simulink model "VCMGCM1962020b_v2"  (R2020b)
settings: Solver=FixedStepDiscrete  StartTime=0.0  StopTime=10.0  FixedStep=0.005  RelTol=1e-3  EnableMultiTasking=on
PreLoadFcn:
  | try, model_open; catch, disp('Error occurred while executing model pre-load callback: model_open.m'); disp('Please assure that the MATLAB working directory is set to the model directory before opening.'); end
InitFcn:
  | try, model_open; catch, end
undefined symbols (not defined in the file): Bridge, GCM, H, raptor_get_param_eval, raptor_get_safe_string, raptor_xcp_function
libraries: Blocks_lib x1165, Raptor_lib x665, simulink x62, VCM_lib x5
(part 10 of 23)

== system VCMGCM1962020b_v2/Fgnd/Diagnostics/Fault Statuses/Drive Cycle Logic/Drive Cycle Complete ==
  WarmUp : Inport
  Enable : EnablePort
  Cntr : Blocks_lib/Cntr  nam='OBDDrvCycleCount'  init=0  inc=1  typ=double  storage=NonVolatile (EEPROM)  use_vardec=on  view_as=Number  enum_struct={}  gain=1  units='count'  help='OBD drive cycle count'  group=group
  Header : Blocks_lib/Header  width=Portrait  addtext=''
  raptor_sfun_obd_driveCycle : Raptor_lib/Faults/OBD/raptor_sfun_obd_driveCycle  Priority=0  inhibitPort=off
      settings: SourceProductName=Raptor
  wires:
  WarmUp/1 -> raptor_sfun_obd_driveCycle/1

== system VCMGCM1962020b_v2/Fgnd/Diagnostics/Fault Statuses/Drive Cycle Logic/Warm-Up ==
  Data : Inport
  Add : Sum  Inputs=+-  InputSameDT=on  OutDataTypeStr=Inherit: Same as first input
  Bus Selector : BusSelector  OutputSignals=VirtualSensors.DrvInvtr.DrvMtrTemp [degC]
  Bus Selector1 : BusSelector  OutputSignals=Control.Mode.StartStop.RunMode [Bool]
  Bus Selector2 : BusSelector  OutputSignals=VirtualSensors.DrvInvtr.DrvMtrTemp [degC]
  Bus Selector3 : BusSelector  OutputSignals=Control.Mode.StartStop.RunMode [Bool]
  Detect Increase : simulink/Logic and Bit Operations/Detect Increase  vinit=0.0  OutDataTypeStr=boolean
  Header : Blocks_lib/Header  width=Portrait  addtext=''
  Hld : Blocks_lib/Hld  init=0
  Logical Operator : Logic  OutDataTypeStr=boolean
  Relational Operator1 : RelationalOperator  OutDataTypeStr=boolean  RndMeth=Nearest  InputSameDT=on
  Relational Operator2 : RelationalOperator  OutDataTypeStr=boolean  RndMeth=Nearest  InputSameDT=on
  SetRst : Blocks_lib/SetRst  init=0
  raptor_adjustment : Raptor_lib/Data Storage/raptor_adjustment  paramName='OBDWarmUpMtrTempDeltaThr'  nameSource=Parameter  initValue=0  dataType=double  storage=Calibration  calDispType=Number  calEnum={'Disabled', 'Enabled'}  calGain=1  calOffset=0  calMax=inf  calMin=-inf  calFormat=''  calUnit='degC'  calHelp='OBD warm-up cycle motor temp delta (from startup) threshold'  calAccess=1  calFunction=group  calDispHeaders=off  calColHeaders={'Col1' 'Col2' 'Col3'}  calRowHeaders={'Row1' 'Row2' 'Row3'}
      settings: SourceProductName=Raptor
  raptor_adjustment2 : Raptor_lib/Data Storage/raptor_adjustment  paramName='OBDWarmUpMtrTempThr'  nameSource=Parameter  initValue=0  dataType=double  storage=Calibration  calDispType=Number  calEnum={'Disabled', 'Enabled'}  calGain=1  calOffset=0  calMax=inf  calMin=-inf  calFormat=''  calUnit='degC'  calHelp='OBD warm-up cycle motor temp threshold'  calAccess=1  calFunction=group  calDispHeaders=off  calColHeaders={'Col1' 'Col2' 'Col3'}  calRowHeaders={'Row1' 'Row2' 'Row3'}
      settings: SourceProductName=Raptor
  raptor_measurement : Raptor_lib/Data Storage/raptor_measurement  paramName='OBDWarmUp'  nameSource=Parameter  calDispType=Number  calEnum={}  calGain=1  calOffset=0  calMax=inf  calMin=-inf  calFormat=''  calUnit='Bool'  calHelp='OBD warm-up achieved'  calAccess=1  calFunction=group  calVisible=on
      settings: SourceProductName=Raptor
  Bool : Outport  VectorParamsAs1DForOutWhenUnconnected=off
  wires:
  Bus Selector3/1 -> Detect Increase/1  "<RunMode [Bool]>"
  Bus Selector2/1 -> Relational Operator1/1  "<DrvMtrTemp [degC]>"
  raptor_adjustment2/1 -> Relational Operator1/2
  Relational Operator1/1 -> Logical Operator/2
  Add/1 -> Relational Operator2/1
  raptor_adjustment/1 -> Relational Operator2/2
  Relational Operator2/1 -> Logical Operator/1
  SetRst/1 -> raptor_measurement/1, Bool/1
  Logical Operator/1 -> SetRst/1
  Detect Increase/1 -> SetRst/2
  Bus Selector/1 -> Hld/2, Add/1  "<DrvMtrTemp [degC]>"
  Data/1 -> Bus Selector3/1, Bus Selector2/1, Bus Selector1/1, Bus Selector/1
  Hld/1 -> Add/2
  Bus Selector1/1 -> Hld/1  "<RunMode [Bool]>"

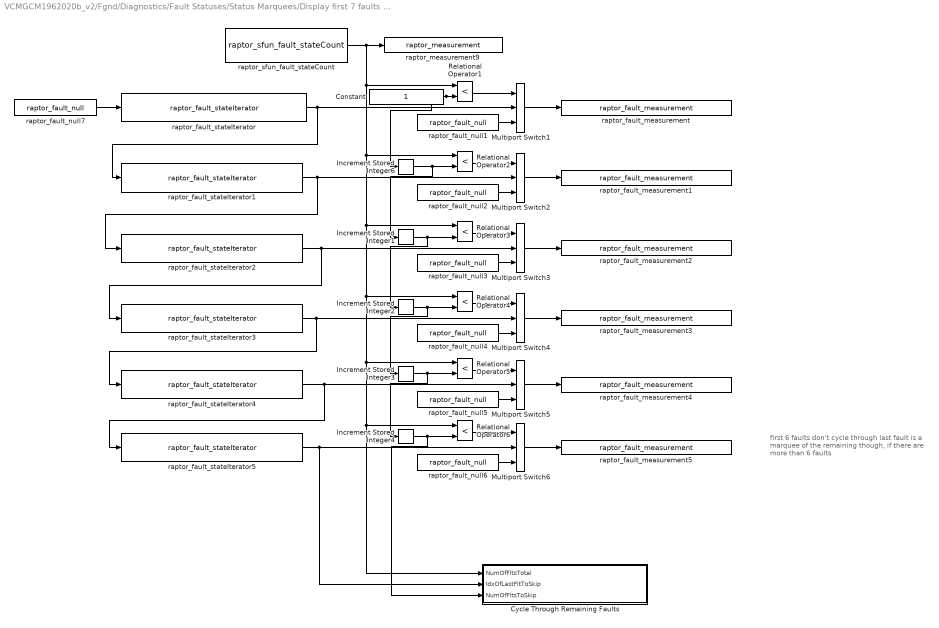
== system VCMGCM1962020b_v2/Fgnd/Diagnostics/Fault Statuses/Status Marquees/Display first 7 faults with the selected state1 ==
  note: first 6 faults don't cycle through
      | last fault is a marquee of the remaining though,
      | if there are more than 6 faults
  Constant : Constant  OutDataTypeStr=Inherit: Inherit via back propagation
  Cycle Through Remaining Faults : Subsystem
  Increment Stored Integer{1..4,6} (5 alike) : simulink/Additional Math & Discrete/Additional Math: Increment - Decrement/Increment Stored Integer
  Multiport Switch{1..6} (6 alike) : MultiPortSwitch  DataPortOrder=Zero-based contiguous  Inputs=2  zeroidx=on
  Relational Operator{1..6} (6 alike) : RelationalOperator  Operator=<  OutDataTypeStr=boolean  RndMeth=Nearest
  raptor_fault_measurement : Raptor_lib/Faults/raptor_fault_measurement  dataName=[finalVarName '1']  calHelp='one of the faults that have failed this drive cycle'  calAccess=1  calFunction=[group ' | ' finalVarName]
      settings: SourceProductName=Raptor
  raptor_fault_measurement1 : Raptor_lib/Faults/raptor_fault_measurement  dataName=[finalVarName '2']  calHelp='one of the faults that have failed this drive cycle'  calAccess=1  calFunction=[group ' | ' finalVarName]
      settings: SourceProductName=Raptor
  raptor_fault_measurement2 : Raptor_lib/Faults/raptor_fault_measurement  dataName=[finalVarName '3']  calHelp='one of the faults that have failed this drive cycle'  calAccess=1  calFunction=[group ' | ' finalVarName]
      settings: SourceProductName=Raptor
  raptor_fault_measurement3 : Raptor_lib/Faults/raptor_fault_measurement  dataName=[finalVarName '4']  calHelp='one of the faults that have failed this drive cycle'  calAccess=1  calFunction=[group ' | ' finalVarName]
      settings: SourceProductName=Raptor
  raptor_fault_measurement4 : Raptor_lib/Faults/raptor_fault_measurement  dataName=[finalVarName '5']  calHelp='one of the faults that have failed this drive cycle'  calAccess=1  calFunction=[group ' | ' finalVarName]
      settings: SourceProductName=Raptor
  raptor_fault_measurement5 : Raptor_lib/Faults/raptor_fault_measurement  dataName=[finalVarName '6']  calHelp='one of the faults that have failed this drive cycle'  calAccess=1  calFunction=[group ' | ' finalVarName]
      settings: SourceProductName=Raptor
  raptor_fault_null{1..7} (7 alike) : Raptor_lib/Faults/raptor_fault_null  null=0
      settings: SourceProductName=Raptor
  raptor_fault_stateIterator{,1..5} (6 alike) : Raptor_lib/Faults/raptor_fault_stateIterator  notOccurred=off  suspected=off  active=off  occurred=off  failedThisDC=off  testCmpltThisDC=off  failing=on  pending=off  confirmed=off  mil=off  permanent=off  ready=off  prevConfirmed=off  failedSinceClear=off  failedLastDC=off  prevMil=off
      settings: SourceProductName=Raptor
  raptor_measurement9 : Raptor_lib/Data Storage/raptor_measurement  paramName=[finalVarName 'Count']  nameSource=Parameter  calDispType=Number  calEnum={'False', 'True'}  calGain=1.0  calOffset=0.0  calMax=inf  calMin=-inf  calFormat='-1'  calUnit=''  calHelp=''  calAccess=1  calFunction=[group ' | ' finalVarName]  calVisible=on
      settings: SourceProductName=Raptor
  raptor_sfun_fault_stateCount : Raptor_lib/Faults/raptor_sfun_fault_stateCount  notOccurred=off  suspected=off  active=off  occurred=off  failedThisDC=off  failing=on  testCmpltThisDC=off  pending=off  confirmed=off  mil=off  permanent=off  ready=off  prevConfirmed=off  failedSinceClear=off  failedLastDC=off  prevMil=off
      settings: SourceProductName=Raptor
  wires:
  Multiport Switch4/1 -> raptor_fault_measurement3/1
  raptor_fault_stateIterator3/1 -> Multiport Switch4/2, raptor_fault_stateIterator4/1
  raptor_fault_null4/1 -> Multiport Switch4/3
  Relational Operator4/1 -> Multiport Switch4/1
  Increment Stored Integer2/1 -> Relational Operator4/2, Increment Stored Integer3/1
  Constant/1 -> Increment Stored Integer6/1, Relational Operator1/2
  Relational Operator1/1 -> Multiport Switch1/1
  raptor_fault_null1/1 -> Multiport Switch1/3
  Multiport Switch1/1 -> raptor_fault_measurement/1
  raptor_sfun_fault_stateCount/1 -> Relational Operator1/1, Relational Operator2/1, Relational Operator3/1, Relational Operator4/1, Relational Operator5/1, Relational Operator6/1, Cycle Through Remaining Faults/1(NumOfFltsTotal), raptor_measurement9/1
  Multiport Switch6/1 -> raptor_fault_measurement5/1
  Relational Operator6/1 -> Multiport Switch6/1
  raptor_fault_stateIterator5/1 -> Multiport Switch6/2, Cycle Through Remaining Faults/2(IdxOfLastFltToSkip)
  Increment Stored Integer4/1 -> Relational Operator6/2, Cycle Through Remaining Faults/3(NumOfFltsToSkip)
  raptor_fault_null6/1 -> Multiport Switch6/3
  Increment Stored Integer3/1 -> Relational Operator5/2, Increment Stored Integer4/1
  raptor_fault_stateIterator/1 -> raptor_fault_stateIterator1/1, Multiport Switch1/2
  Relational Operator2/1 -> Multiport Switch2/1
  raptor_fault_null2/1 -> Multiport Switch2/3
  raptor_fault_null7/1 -> raptor_fault_stateIterator/1
  Relational Operator5/1 -> Multiport Switch5/1
  raptor_fault_stateIterator4/1 -> Multiport Switch5/2, raptor_fault_stateIterator5/1
  Multiport Switch5/1 -> raptor_fault_measurement4/1
  raptor_fault_null5/1 -> Multiport Switch5/3
  raptor_fault_stateIterator1/1 -> Multiport Switch2/2, raptor_fault_stateIterator2/1
  Multiport Switch2/1 -> raptor_fault_measurement1/1
  Multiport Switch3/1 -> raptor_fault_measurement2/1
  raptor_fault_stateIterator2/1 -> Multiport Switch3/2, raptor_fault_stateIterator3/1
  Relational Operator3/1 -> Multiport Switch3/1
  Increment Stored Integer6/1 -> Relational Operator2/2, Increment Stored Integer1/1
  raptor_fault_null3/1 -> Multiport Switch3/3
  Increment Stored Integer1/1 -> Relational Operator3/2, Increment Stored Integer2/1

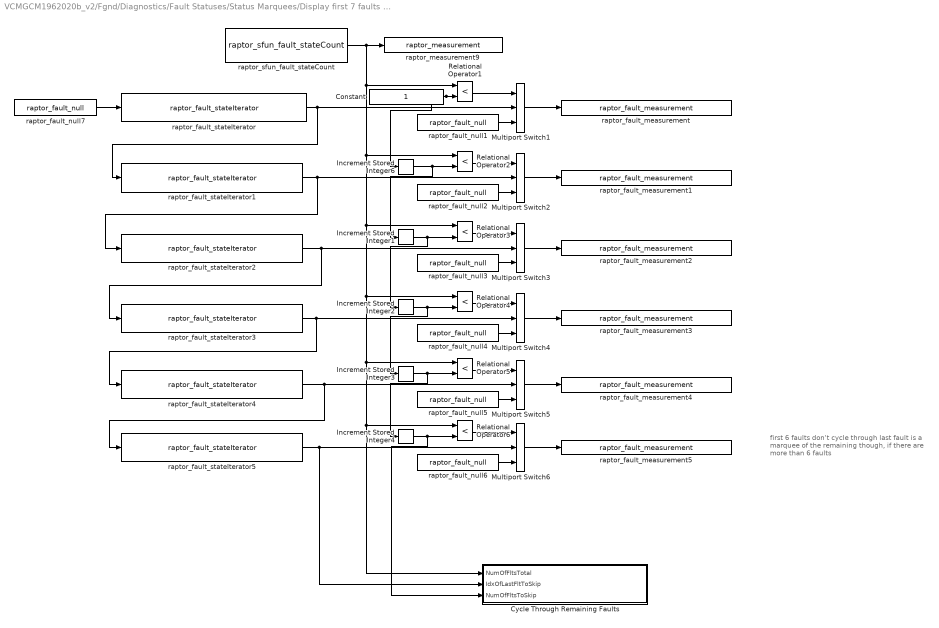
== system VCMGCM1962020b_v2/Fgnd/Diagnostics/Fault Statuses/Status Marquees/Display first 7 faults with the selected state2 ==
  note: first 6 faults don't cycle through
      | last fault is a marquee of the remaining though,
      | if there are more than 6 faults
  Constant : Constant  OutDataTypeStr=Inherit: Inherit via back propagation
  Cycle Through Remaining Faults : Subsystem
  Increment Stored Integer{1..4,6} (5 alike) : simulink/Additional Math & Discrete/Additional Math: Increment - Decrement/Increment Stored Integer
  Multiport Switch{1..6} (6 alike) : MultiPortSwitch  DataPortOrder=Zero-based contiguous  Inputs=2  zeroidx=on
  Relational Operator{1..6} (6 alike) : RelationalOperator  Operator=<  OutDataTypeStr=boolean  RndMeth=Nearest
  raptor_fault_measurement : Raptor_lib/Faults/raptor_fault_measurement  dataName=[finalVarName '1']  calHelp='one of the faults that have failed this drive cycle'  calAccess=1  calFunction=[group ' | ' finalVarName]
      settings: SourceProductName=Raptor
  raptor_fault_measurement1 : Raptor_lib/Faults/raptor_fault_measurement  dataName=[finalVarName '2']  calHelp='one of the faults that have failed this drive cycle'  calAccess=1  calFunction=[group ' | ' finalVarName]
      settings: SourceProductName=Raptor
  raptor_fault_measurement2 : Raptor_lib/Faults/raptor_fault_measurement  dataName=[finalVarName '3']  calHelp='one of the faults that have failed this drive cycle'  calAccess=1  calFunction=[group ' | ' finalVarName]
      settings: SourceProductName=Raptor
  raptor_fault_measurement3 : Raptor_lib/Faults/raptor_fault_measurement  dataName=[finalVarName '4']  calHelp='one of the faults that have failed this drive cycle'  calAccess=1  calFunction=[group ' | ' finalVarName]
      settings: SourceProductName=Raptor
  raptor_fault_measurement4 : Raptor_lib/Faults/raptor_fault_measurement  dataName=[finalVarName '5']  calHelp='one of the faults that have failed this drive cycle'  calAccess=1  calFunction=[group ' | ' finalVarName]
      settings: SourceProductName=Raptor
  raptor_fault_measurement5 : Raptor_lib/Faults/raptor_fault_measurement  dataName=[finalVarName '6']  calHelp='one of the faults that have failed this drive cycle'  calAccess=1  calFunction=[group ' | ' finalVarName]
      settings: SourceProductName=Raptor
  raptor_fault_null{1..7} (7 alike) : Raptor_lib/Faults/raptor_fault_null  null=0
      settings: SourceProductName=Raptor
  raptor_fault_stateIterator{,1..5} (6 alike) : Raptor_lib/Faults/raptor_fault_stateIterator  notOccurred=off  suspected=off  active=off  occurred=off  failedThisDC=on  testCmpltThisDC=off  failing=off  pending=off  confirmed=off  mil=off  permanent=off  ready=off  prevConfirmed=off  failedSinceClear=off  failedLastDC=off  prevMil=off
      settings: SourceProductName=Raptor
  raptor_measurement9 : Raptor_lib/Data Storage/raptor_measurement  paramName=[finalVarName 'Count']  nameSource=Parameter  calDispType=Number  calEnum={'False', 'True'}  calGain=1.0  calOffset=0.0  calMax=inf  calMin=-inf  calFormat='-1'  calUnit=''  calHelp=''  calAccess=1  calFunction=[group ' | ' finalVarName]  calVisible=on
      settings: SourceProductName=Raptor
  raptor_sfun_fault_stateCount : Raptor_lib/Faults/raptor_sfun_fault_stateCount  notOccurred=off  suspected=off  active=off  occurred=off  failedThisDC=on  failing=off  testCmpltThisDC=off  pending=off  confirmed=off  mil=off  permanent=off  ready=off  prevConfirmed=off  failedSinceClear=off  failedLastDC=off  prevMil=off
      settings: SourceProductName=Raptor
  wires:
  Increment Stored Integer1/1 -> Increment Stored Integer2/1, Relational Operator3/2
  raptor_fault_null3/1 -> Multiport Switch3/3
  Increment Stored Integer6/1 -> Increment Stored Integer1/1, Relational Operator2/2
  Relational Operator3/1 -> Multiport Switch3/1
  raptor_fault_stateIterator2/1 -> raptor_fault_stateIterator3/1, Multiport Switch3/2
  Multiport Switch3/1 -> raptor_fault_measurement2/1
  Multiport Switch2/1 -> raptor_fault_measurement1/1
  raptor_fault_stateIterator1/1 -> raptor_fault_stateIterator2/1, Multiport Switch2/2
  raptor_fault_null5/1 -> Multiport Switch5/3
  Multiport Switch5/1 -> raptor_fault_measurement4/1
  raptor_fault_stateIterator4/1 -> raptor_fault_stateIterator5/1, Multiport Switch5/2
  Relational Operator5/1 -> Multiport Switch5/1
  raptor_fault_null7/1 -> raptor_fault_stateIterator/1
  raptor_fault_null2/1 -> Multiport Switch2/3
  Relational Operator2/1 -> Multiport Switch2/1
  raptor_fault_stateIterator/1 -> Multiport Switch1/2, raptor_fault_stateIterator1/1
  Increment Stored Integer3/1 -> Increment Stored Integer4/1, Relational Operator5/2
  raptor_fault_null6/1 -> Multiport Switch6/3
  Increment Stored Integer4/1 -> Cycle Through Remaining Faults/3(NumOfFltsToSkip), Relational Operator6/2
  raptor_fault_stateIterator5/1 -> Cycle Through Remaining Faults/2(IdxOfLastFltToSkip), Multiport Switch6/2
  Relational Operator6/1 -> Multiport Switch6/1
  Multiport Switch6/1 -> raptor_fault_measurement5/1
  raptor_sfun_fault_stateCount/1 -> raptor_measurement9/1, Cycle Through Remaining Faults/1(NumOfFltsTotal), Relational Operator6/1, Relational Operator5/1, Relational Operator4/1, Relational Operator3/1, Relational Operator2/1, Relational Operator1/1
  Multiport Switch1/1 -> raptor_fault_measurement/1
  raptor_fault_null1/1 -> Multiport Switch1/3
  Relational Operator1/1 -> Multiport Switch1/1
  Constant/1 -> Relational Operator1/2, Increment Stored Integer6/1
  Increment Stored Integer2/1 -> Increment Stored Integer3/1, Relational Operator4/2
  Relational Operator4/1 -> Multiport Switch4/1
  raptor_fault_null4/1 -> Multiport Switch4/3
  raptor_fault_stateIterator3/1 -> raptor_fault_stateIterator4/1, Multiport Switch4/2
  Multiport Switch4/1 -> raptor_fault_measurement3/1

== system VCMGCM1962020b_v2/Fgnd/Diagnostics/Fault Statuses/Status Marquees/Fault Fail Time ==
  Idx : Inport
  f : TriggerPort  TriggerType=function-call  VariantControl=(inherit)
  Header : Blocks_lib/Header  width=Portrait  addtext=''
  raptor_fault_data_def : Raptor_lib/Faults/raptor_fault_data_def  dataName='FaultFailTime'  initValue=0  dataType=double  storage=Volatile (RAM)  calVisible=off  calType=Measurement  calDispType=Number  calEnum={'Disabled', 'Enabled'}  calGain=1  calOffset=0  calMax=inf  calMin=-inf  calFormat=''  calUnit='count'  calHelp='Fault occurence count'  calAccess=1
      settings: SourceProductName=Raptor
  raptor_fault_data_write : Raptor_lib/Faults/raptor_fault_data_write  dataName='FaultFailTime'  faultSource=Port  faultName='myFaultName'
      settings: SourceProductName=Raptor
  raptor_time : Raptor_lib/Triggers/raptor_time  unit=seconds
      settings: SourceProductName=Raptor
  wires:
  raptor_time/1 -> raptor_fault_data_write/1
  Idx/1 -> raptor_fault_data_write/2

== system VCMGCM1962020b_v2/Fgnd/Sensors/CAN/Battery/BMS1_Currents ==
  note: The signal name says continuous but the dbc file says max current limit
  DiagEnbl : Inport
  Bus Creator : BusCreator  Inputs=5
  CANRxField{1..4} (4 alike) : Blocks_lib/CANRxField  typ='double'  custom=off  custom_nam='---'  custom_units='---'
  CANRxMsgStatus : Blocks_lib/CANRxMsgStatus  samptime=samptime  custom=off  custom_nam='---'  msgnam=BMS1_Currents
      link override CntrSat/Constant: OutDataTypeStr=uint32
      link override CntrSat/Constant1: OutDataTypeStr=uint32
      link override CntrSat/Relational Operator: Operator=>
      link override CntrSat/raptor_adjustment: dataType=uint32
  Header : Blocks_lib/Header  width=Landscape  addtext=''
  raptor_can_rxmsg : Raptor_lib/CAN/raptor_can_rxmsg  canDefinition=struct('dbcFile', 'eMatrix_Battery.dbc','message', 'BMS1_Currents','comment', '','signals', {{'I_CHG_Cont','I_BAT','I_DCHG_Max','I_CHG_Max'}},'enabled', [ 1 1 1 1;],'scaled', [ 1 1 1 1;],'canBus', '''CAN1''','messageID', [ 273;],'idMask', [ 536870911;],'payloadMask', [],'payloadValue', [],'period', [ 0;],'mailbox', '''''','queueSize', [ 1;],'label', [ 0;],'ver', [ 2;],'showID', [ 0;],'showRaw', [ 0;],'fill', [ 0;],'editID', [ 0;],'signalOrder', [ 3;],'signalAscDes', [ 1;])  canBus='CAN1'  mailbox=''  payloadMask=[]  payloadValue=[]  idMask=hex2dec('1FFFFFFF')  queueSize=1  showID=0  label=0  fill=0  id=273  showRaw=0  showAge=1  signalOrder=3  signalInfo={{struct('Name', 'I_CHG_Cont','Startbit', [ 0;],'SignalSize', [ 16;],'ByteOrder', 'LittleEndian','ValueType', 'UNSIGNED','Class', 'uint16','Signed', [ 0;],'Factor', [ 0.1;],'Offset', [ 0;],'Min', [ 0;],'Max', [ 0;],'Units', 'A','Comment', 'Maximum Charge Current Limit','StartBit', [ 48;]),struct('Name', 'I_BAT','Startbit', [ 0;],'SignalSize', [ 16;],'ByteOrder', 'LittleEndian','ValueType', 'UNSIGNED','Class', 'uint16','Signed', [ 0;],'Factor', [ 0.1;],'Offset', [ 0;],'Min', [ 0;],'Max', [ 0;],'Units', 'A','Comment', 'Total Battery Current (Charge:+, discharge:-)','StartBit', [ 0;]),struct('Name', 'I_DCHG_Max','Startbit', [ 0;],'SignalSize', [ 16;],'ByteOrder', 'LittleEndian','ValueType', 'UNSIGNED','Class', 'uint16','Signed', [ 0;],'Factor', [ 0.1;],'Offset', [ 0;],'Min', [ 0;],'Max', [ 0;],'Units', 'A','Comment', 'Maximum Discharge Current Limit','StartBit', [ 32;]),struct('Name', 'I_CHG_Max','Startbit', [ 0;],'SignalSize', [ 16;],'ByteOrder', 'LittleEndian','ValueType', 'UNSIGNED','Class', 'uint16','Signed', [ 0;],'Factor', [ 0.1;],'Offset', [ 0;],'Min', [ 0;],'Max', [ 0;],'Units', 'A','Comment', 'Maximum Charge Current Limit','StartBit', [ 16;])}}
      settings: SourceProductName=Raptor
  Data : Outport  VectorParamsAs1DForOutWhenUnconnected=off
  wires:
  Bus Creator/1 -> Data/1  "BMS1_Currents"
  CANRxField2/1 -> Bus Creator/3
  CANRxField3/1 -> Bus Creator/4
  CANRxField4/1 -> Bus Creator/5
  raptor_can_rxmsg/2 -> CANRxField1/1  "Batt_CrntCHG_Cont"
  raptor_can_rxmsg/4 -> CANRxField3/1  "Batt_CrntDCHG_Max"
  raptor_can_rxmsg/5 -> CANRxField4/1  "Batt_CrntCHRG_Max"
  CANRxField1/1 -> Bus Creator/2
  CANRxMsgStatus/1 -> Bus Creator/1
  DiagEnbl/1 -> CANRxMsgStatus/1
  raptor_can_rxmsg/1 -> CANRxMsgStatus/2  "Age"
  raptor_can_rxmsg/3 -> CANRxField2/1  "Batt_Current"

== system VCMGCM1962020b_v2/Fgnd/Sensors/CAN/Battery/BMS2_VoltageSOC ==
  DiagEnbl : Inport
  Bus Creator : BusCreator  Inputs=6
  CANRxField{,1..4} (5 alike) : Blocks_lib/CANRxField  typ='double'  custom=off  custom_nam='---'  custom_units='---'
  CANRxMsgStatus : Blocks_lib/CANRxMsgStatus  samptime=samptime  custom=off  custom_nam='---'  msgnam=BMS2_VoltageSOC
      link override CntrSat/Constant: OutDataTypeStr=uint32
      link override CntrSat/Constant1: OutDataTypeStr=uint32
      link override CntrSat/Relational Operator: Operator=>
      link override CntrSat/raptor_adjustment: dataType=uint32
  Header : Blocks_lib/Header  width=Landscape  addtext=''
  raptor_can_rxmsg : Raptor_lib/CAN/raptor_can_rxmsg  canDefinition=struct('dbcFile', 'eMatrix_Battery.dbc','message', 'BMS2_VoltageSOC','comment', '','signals', {{'PackDischargeResistance','PackChargeResistance','SOH','V_BAT','SOC'}},'enabled', [ 1 1 1 1 1;],'scaled', [ 1 1 1 1 1;],'canBus', '''CAN1''','messageID', [ 274;],'idMask', [ 536870911;],'payloadMask', [],'payloadValue', [],'period', [ 0;],'mailbox', '''''','queueSize', [ 1;],'label', [ 0;],'ver', [ 2;],'showID', [ 0;],'showRaw', [ 0;],'fill', [ 0;],'editID', [ 0;],'signalOrder', [ 3;],'signalAscDes', [ 1;])  canBus='CAN1'  mailbox=''  payloadMask=[]  payloadValue=[]  idMask=hex2dec('1FFFFFFF')  queueSize=1  showID=0  label=0  fill=0  id=274  showRaw=0  showAge=1  signalOrder=3  signalInfo={{struct('Name', 'PackDischargeResistance','Startbit', [ 0;],'SignalSize', [ 16;],'ByteOrder', 'LittleEndian','ValueType', 'UNSIGNED','Class', 'uint16','Signed', [ 0;],'Factor', [ 0.0001;],'Offset', [ 0;],'Min', [ 0;],'Max', [ 0;],'Units', 'Ohm','Comment', 'Instantaneous estimated internal resistance of a pack. All packs are calculated and this is the average of all active packs.','StartBit', [ 16;]),struct('Name', 'PackChargeResistance','Startbit', [ 0;],'SignalSize', [ 16;],'ByteOrder', 'LittleEndian','ValueType', 'UNSIGNED','Class', 'uint16','Signed', [ 0;],'Factor', [ 0.0001;],'Offset', [ 0;],'Min', [ 0;],'Max', [ 0;],'Units', 'Ohm','Comment', 'Instantaneous estimated internal resistance of a pack. All packs are calculated and this is the average of all active packs.','StartBit', [ 0;]),struct('Name', 'SOH','Startbit', [ 0;],'SignalSize', [ 8;],'ByteOrder', 'LittleEndian','ValueType', 'UNSIGNED','Class', 'uint8','Signed', [ 0;],'Factor', [ 0.4;],'Offset', [ 0;],'Min', [ 0;],'Max', [ 100;],'Units', '%','Comment', 'State of health.','StartBit', [ 56;]),struct('Name', 'V_BAT','Startbit', [ 0;],'SignalSize', [ 16;],'ByteOrder', 'LittleEndian','ValueType', 'UNSIGNED','Class', 'uint16','Signed', [ 0;],'Factor', [ 0.1;],'Offset', [ 0;],'Min', [ 0;],'Max', [ 450;],'Units', 'V','Comment', 'Total Battery Voltage','StartBit', [ 32;]),struct('Name', 'SOC','Startbit', [ 0;],'SignalSize', [ 8;],'ByteOrder', 'LittleEndian','ValueType', 'UNSIGNED','Class', 'uint8','Signed', [ 0;],'Factor', [ 0.4;],'Offset', [ 0;],'Min', [ 0;],'Max', [ 100;],'Units', '%','Comment', 'State of Charge.','StartBit', [ 48;])}}
      settings: SourceProductName=Raptor
  Data : Outport  VectorParamsAs1DForOutWhenUnconnected=off
  wires:
  raptor_can_rxmsg/1 -> CANRxMsgStatus/2  "Age"
  DiagEnbl/1 -> CANRxMsgStatus/1
  CANRxMsgStatus/1 -> Bus Creator/1
  CANRxField1/1 -> Bus Creator/2
  raptor_can_rxmsg/5 -> CANRxField4/1  "Batt_Volt"
  raptor_can_rxmsg/4 -> CANRxField3/1  "Batt_SOH"
  raptor_can_rxmsg/3 -> CANRxField2/1  "Batt_CHG_Res"
  raptor_can_rxmsg/2 -> CANRxField1/1  "Batt_DCHG_Res"
  CANRxField4/1 -> Bus Creator/5
  CANRxField3/1 -> Bus Creator/4
  CANRxField2/1 -> Bus Creator/3
  Bus Creator/1 -> Data/1  "BMS2_VoltageSOC"
  raptor_can_rxmsg/6 -> CANRxField/1  "Batt_SOC"
  CANRxField/1 -> Bus Creator/6

== system VCMGCM1962020b_v2/Fgnd/Sensors/CAN/Battery/BMS3_Cell ==
  DiagEnbl : Inport
  Bus Creator : BusCreator  Inputs=6
  CANRxField{,1,3..4} (4 alike) : Blocks_lib/CANRxField  typ='double'  custom=off  custom_nam='---'  custom_units='---'
  CANRxField2 : Blocks_lib/CANRxField  typ='uint8'  custom=off  custom_nam='---'  custom_units='---'
  CANRxMsgStatus : Blocks_lib/CANRxMsgStatus  samptime=samptime  custom=off  custom_nam='---'  msgnam=BMS3_Cell
      link override CntrSat/Constant: OutDataTypeStr=uint32
      link override CntrSat/Constant1: OutDataTypeStr=uint32
      link override CntrSat/Relational Operator: Operator=>
      link override CntrSat/raptor_adjustment: dataType=uint32
  Header : Blocks_lib/Header  width=Landscape  addtext=''
  raptor_can_rxmsg : Raptor_lib/CAN/raptor_can_rxmsg  canDefinition=struct('dbcFile', 'eMatrix_Battery.dbc','message', 'BMS3_Cell','comment', '','signals', {{'Vest_Avg','T_Cell_Min','T_Cell_Max','V_Cell_Min','V_Cell_Max'}},'enabled', [ 1 1 1 1 1;],'scaled', [ 1 1 1 1 1;],'canBus', '''CAN1''','messageID', [ 275;],'idMask', [ 536870911;],'payloadMask', [],'payloadValue', [],'period', [ 0;],'mailbox', '''''','queueSize', [ 1;],'label', [ 0;],'ver', [ 2;],'showID', [ 0;],'showRaw', [ 0;],'fill', [ 0;],'editID', [ 0;],'signalOrder', [ 3;],'signalAscDes', [ 1;])  canBus='CAN1'  mailbox=''  payloadMask=[]  payloadValue=[]  idMask=hex2dec('1FFFFFFF')  queueSize=1  showID=0  label=0  fill=0  id=275  showRaw=0  showAge=1  signalOrder=3  signalInfo={{struct('Name', 'Vest_Avg','Startbit', [ 0;],'SignalSize', [ 16;],'ByteOrder', 'LittleEndian','ValueType', 'UNSIGNED','Class', 'uint16','Signed', [ 0;],'Factor', [ 0.001;],'Offset', [ 0;],'Min', [ 0;],'Max', [ 10;],'Units', 'V','Comment', 'Estimated terminal voltage based on average cell voltage.','StartBit', [ 48;]),struct('Name', 'T_Cell_Min','Startbit', [ 0;],'SignalSize', [ 8;],'ByteOrder', 'LittleEndian','ValueType', 'UNSIGNED','Class', 'uint8','Signed', [ 0;],'Factor', [ 0.5;],'Offset', [ -40;],'Min', [ -40;],'Max', [ 87.5;],'Units', 'C','Comment', 'Minimum Cell Temperature','StartBit', [ 40;]),struct('Name', 'T_Cell_Max','Startbit', [ 0;],'SignalSize', [ 8;],'ByteOrder', 'LittleEndian','ValueType', 'UNSIGNED','Class', 'uint8','Signed', [ 0;],'Factor', [ 0.5;],'Offset', [ -40;],'Min', [ -40;],'Max', [ 87.5;],'Units', 'C','Comment', 'Maximum cell Temperature','StartBit', [ 32;]),struct('Name', 'V_Cell_Min','Startbit', [ 0;],'SignalSize', [ 16;],'ByteOrder', 'LittleEndian','ValueType', 'UNSIGNED','Class', 'uint16','Signed', [ 0;],'Factor', [ 0.001;],'Offset', [ 0;],'Min', [ 0;],'Max', [ 10;],'Units', 'V','Comment', 'Instantaneous minimum cell voltage.','StartBit', [ 16;]),struct('Name', 'V_Cell_Max','Startbit', [ 0;],'SignalSize', [ 16;],'ByteOrder', 'LittleEndian','ValueType', 'UNSIGNED','Class', 'uint16','Signed', [ 0;],'Factor', [ 0.001;],'Offset', [ 0;],'Min', [ 0;],'Max', [ 10;],'Units', 'V','Comment', 'Instantaneous maximum Cell voltage.','StartBit', [ 0;])}}
      settings: SourceProductName=Raptor
  Data : Outport  VectorParamsAs1DForOutWhenUnconnected=off
  wires:
  raptor_can_rxmsg/1 -> CANRxMsgStatus/2  "Age"
  DiagEnbl/1 -> CANRxMsgStatus/1
  CANRxMsgStatus/1 -> Bus Creator/1
  CANRxField1/1 -> Bus Creator/2
  raptor_can_rxmsg/5 -> CANRxField3/1  "Batt_Volt_CellMin"
  raptor_can_rxmsg/4 -> CANRxField/1  "Batt_Temp_CellMax"
  raptor_can_rxmsg/3 -> CANRxField2/1  "Batt_Temp_CellMin"
  raptor_can_rxmsg/2 -> CANRxField1/1  "Batt_VestAvg"
  CANRxField3/1 -> Bus Creator/5
  CANRxField/1 -> Bus Creator/4
  CANRxField2/1 -> Bus Creator/3
  Bus Creator/1 -> Data/1  "BMS3_Cell"
  raptor_can_rxmsg/6 -> CANRxField4/1  "Batt_Volt_CellMax"
  CANRxField4/1 -> Bus Creator/6

== system VCMGCM1962020b_v2/Fgnd/Sensors/CAN/Battery/BMS4_MasterStatus ==
  DiagEnbl : Inport
  Bus Creator : BusCreator  Inputs=13
  CANRxField1 : Blocks_lib/CANRxField  typ='double'  custom=off  custom_nam='---'  custom_units='---'
  CANRxField{3..12} (10 alike) : Blocks_lib/CANRxField  typ='boolean'  custom=off  custom_nam='---'  custom_units='---'
  CANRxField2 : Blocks_lib/CANRxField  typ='uint8'  custom=off  custom_nam='---'  custom_units='---'
  CANRxMsgStatus : Blocks_lib/CANRxMsgStatus  samptime=samptime  custom=off  custom_nam='---'  msgnam=BMS4_MasterStatus
      link override CntrSat/Constant: OutDataTypeStr=uint32
      link override CntrSat/Constant1: OutDataTypeStr=uint32
      link override CntrSat/Relational Operator: Operator=>
      link override CntrSat/raptor_adjustment: dataType=uint32
  Header : Blocks_lib/Header  width=Landscape  addtext=''
  raptor_can_rxmsg : Raptor_lib/CAN/raptor_can_rxmsg  canDefinition=struct('dbcFile', 'eMatrix_Battery.dbc','message', 'BMS4_MasterStatus','comment', '','signals', {{'NumberOfPacks','kWhThroughput','kWh','CoolantTemp','HVIL','MainContactorStep','StartInhibit','MIL','FaultActive','MainContactorStatus','FAN_Fb','Balancing'}},'enabled', [ 1 1 1 1 1 1 1 1 1 1 1 1;],'scaled', [ 1 1 1 1 1 1 1 1 1 1 1 1;],'canBus', '''CAN1''','messageID', [ 276;],'idMask', [ 536870911;],'payloadMask', [],'payloadValue', [],'period', [ 0;],'mailbox', '''''','queueSize', [ 1;],'label', [ 0;],'ver', [ 2;],'showID', [ 0;],'showRaw', [ 0;],'fill', [ 0;],'editID', [ 0;],'signalOrder', [ 3;],'signalAscDes', [ 1;])  canBus='CAN1'  mailbox=''  payloadMask=[]  payloadValue=[]  idMask=hex2dec('1FFFFFFF')  queueSize=1  showID=0  label=0  fill=0  id=276  showRaw=0  showAge=1  signalOrder=3  signalInfo={{struct('Name', 'NumberOfPacks','Startbit', [ 0;],'SignalSize', [ 3;],'ByteOrder', 'LittleEndian','ValueType', 'UNSIGNED','Class', 'uint8','Signed', [ 0;],'Factor', [ 1;],'Offset', [ 0;],'Min', [ 0;],'Max', [ 0;],'Units', '','Comment', '','StartBit', [ 61;]),struct('Name', 'kWhThroughput','Startbit', [ 0;],'SignalSize', [ 21;],'ByteOrder', 'LittleEndian','ValueType', 'UNSIGNED','Class', 'uint32','Signed', [ 0;],'Factor', [ 1;],'Offset', [ 0;],'Min', [ 0;],'Max', [ 2097151;],'Units', 'kWh','Comment', 'integral of absolute value of power measured at the battery terminals.','StartBit', [ 40;]),struct('Name', 'kWh','Startbit', [ 0;],'SignalSize', [ 16;],'ByteOrder', 'LittleEndian','ValueType', 'UNSIGNED','Class', 'uint16','Signed', [ 0;],'Factor', [ 0.001;],'Offset', [ 0;],'Min', [ 0;],'Max', [ 0;],'Units', 'kWh','Comment', 'Integral of power measured at the battery.','StartBit', [ 24;]),struct('Name', 'CoolantTemp','Startbit', [ 0;],'SignalSize', [ 8;],'ByteOrder', 'LittleEndian','ValueType', 'UNSIGNED','Class', 'uint8','Signed', [ 0;],'Factor', [ 0.5;],'Offset', [ -40;],'Min', [ -40;],'Max', [ 87.5;],'Units', 'C','Comment', 'Air side coolant temperature.','StartBit', [ 16;]),struct('Name', 'HVIL','Startbit', [ 0;],'SignalSize', [ 1;],'ByteOrder', 'LittleEndian','ValueType', 'UNSIGNED','Class', 'uint8','Signed', [ 0;],'Factor', [ 1;],'Offset', [ 0;],'Min', [ 0;],'Max', [ 1;],'Units', 'Bool ','Comment', '1 = HVIL circuit closed','StartBit', [ 14;]),struct('Name', 'MainContactorStep','Startbit', [ 0;],'SignalSize', [ 8;],'ByteOrder', 'LittleEndian','ValueType', 'SIGNED','Class', 'int8','Signed', [ 1;],'Factor', [ 1;],'Offset', [ 0;],'Min', [ 0;],'Max', [ 0;],'Units', 'Enum','Comment', 'Startup and shutdown state. Positive values are startup and negative values are shutdown.','StartBit', [ 0;]),struct('Name', 'StartInhibit','Startbit', [ 0;],'SignalSize', [ 1;],'ByteOrder', 'LittleEndian','ValueType', 'UNSIGNED','Class', 'uint8','Signed', [ 0;],'Factor', [ 1;],'Offset', [ 0;],'Min', [ 0;],'Max', [ 1;],'Units', 'Bool ','Comment', 'Vehicle Start Inhibit Request. If this is 1 then some malfunction is preventing the battery from providing current.','StartBit', [ 9;]),struct('Name', 'MIL','Startbit', [ 0;],'SignalSize', [ 1;],'ByteOrder', 'LittleEndian','ValueType', 'UNSIGNED','Class', 'uint8','Signed', [ 0;],'Factor', [ 1;],'Offset', [ 0;],'Min', [ 0;],'Max', [ 1;],'Units', 'Bool ','Comment', 'Service Request.','StartBit', [ 10;]),struct('Name', 'FaultActive','Startbit', [ 0;],'SignalSize', [ 1;],'ByteOrder', 'LittleEndian','ValueType', 'UNSIGNED','Class', 'uint8','Signed', [ 0;],'Factor', [ 1;],'Offset', [ 0;],'Min', [ 0;],'Max', [ 1;],'Units', 'Bool ','Comment', 'Malfunction indicator lamp.','StartBit', [ 11;]),struct('Name', 'MainContactorStatus','Startbit', [ 0;],'SignalSize', [ 1;],'ByteOrder', 'LittleEndian','ValueType', 'UNSIGNED','Class', 'uint8','Signed', [ 0;],'Factor', [ 1;],'Offset', [ 0;],'Min', [ 0;],'Max', [ 0;],'Units', 'Bool ','Comment', 'logical status. If status is 1 then the battery can provide current. If 0 then the vehicle should not try to draw current.','StartBit', [ 8;]),struct('Name', 'FAN_Fb','Startbit', [ 0;],'SignalSize', [ 1;],'ByteOrder', 'LittleEndian','ValueType', 'UNSIGNED','Class', 'uint8','Signed', [ 0;],'Factor', [ 1;],'Offset', [ 0;],'Min', [ 0;],'Max', [ 1;],'Units', 'Bool ','Comment', 'Heating or Cooling Fan ON feedback','StartBit', [ 13;]),struct('Name', 'Balancing','Startbit', [ 0;],'SignalSize', [ 1;],'ByteOrder', 'LittleEndian','ValueType', 'UNSIGNED','Class', 'uint8','Signed', [ 0;],'Factor', [ 1;],'Offset', [ 0;],'Min', [ 0;],'Max', [ 1;],'Units', 'Bool ','Comment', 'Battery Cell balancing state.','StartBit', [ 12;])}}
      settings: SourceProductName=Raptor
  Data : Outport  VectorParamsAs1DForOutWhenUnconnected=off
  wires:
  Bus Creator/1 -> Data/1  "BMS4_MasterStatus"
  CANRxField2/1 -> Bus Creator/3
  CANRxField3/1 -> Bus Creator/4
  CANRxField4/1 -> Bus Creator/5
  raptor_can_rxmsg/2 -> CANRxField1/1  "Batt_NmbrPcks"
  raptor_can_rxmsg/3 -> CANRxField2/1  "Batt_kWhThroughput"
  raptor_can_rxmsg/4 -> CANRxField3/1  "Batt_kWh"
  raptor_can_rxmsg/5 -> CANRxField4/1  "Batt_CoolntTemp"
  CANRxField1/1 -> Bus Creator/2
  CANRxMsgStatus/1 -> Bus Creator/1
  DiagEnbl/1 -> CANRxMsgStatus/1
  raptor_can_rxmsg/1 -> CANRxMsgStatus/2  "Age"
  raptor_can_rxmsg/6 -> CANRxField5/1  "Batt_HVIL"
  CANRxField5/1 -> Bus Creator/6
  raptor_can_rxmsg/7 -> CANRxField6/1  "Batt_MnCntcrStp"
  CANRxField6/1 -> Bus Creator/7
  raptor_can_rxmsg/8 -> CANRxField7/1  "Batt_StartInhibit"
  CANRxField7/1 -> Bus Creator/8
  raptor_can_rxmsg/9 -> CANRxField8/1  "Batt_SrvcRqst"
  CANRxField8/1 -> Bus Creator/9
  raptor_can_rxmsg/10 -> CANRxField9/1  "Batt_Fault"
  CANRxField9/1 -> Bus Creator/10
  raptor_can_rxmsg/11 -> CANRxField10/1  "Batt_MainCntctrStatus"
  CANRxField10/1 -> Bus Creator/11
  raptor_can_rxmsg/12 -> CANRxField11/1  "Batt_Fan"
  CANRxField11/1 -> Bus Creator/12
  raptor_can_rxmsg/13 -> CANRxField12/1  "Batt_Balancing_Sts"
  CANRxField12/1 -> Bus Creator/13

== system VCMGCM1962020b_v2/Fgnd/Sensors/CAN/Battery/BMS6_Energy ==
  DiagEnbl : Inport
  Bus Creator : BusCreator  Inputs=2
  CANRxField1 : Blocks_lib/CANRxField  typ='double'  custom=off  custom_nam='---'  custom_units='---'
  CANRxMsgStatus : Blocks_lib/CANRxMsgStatus  samptime=samptime  custom=off  custom_nam='---'  msgnam=BMS6_Energy
      link override CntrSat/Constant: OutDataTypeStr=uint32
      link override CntrSat/Constant1: OutDataTypeStr=uint32
      link override CntrSat/Relational Operator: Operator=>
      link override CntrSat/raptor_adjustment: dataType=uint32
  Header : Blocks_lib/Header  width=Landscape  addtext=''
  raptor_can_rxmsg : Raptor_lib/CAN/raptor_can_rxmsg  canDefinition=struct('dbcFile', 'eMatrix_Battery.dbc','message', 'BMS6_Energy','comment', '','signals', {{'EnergyRemaining'}},'enabled', [ 1;],'scaled', [ 1;],'canBus', '''CAN1''','messageID', [ 278;],'idMask', [ 536870911;],'payloadMask', [],'payloadValue', [],'period', [ 0;],'mailbox', '''''','queueSize', [ 1;],'label', [ 0;],'ver', [ 2;],'showID', [ 0;],'showRaw', [ 0;],'fill', [ 0;],'editID', [ 0;],'signalOrder', [ 3;],'signalAscDes', [ 1;])  canBus='CAN1'  mailbox=''  payloadMask=[]  payloadValue=[]  idMask=hex2dec('1FFFFFFF')  queueSize=1  showID=0  label=0  fill=0  id=278  showRaw=0  showAge=1  signalOrder=3  signalInfo={{struct('Name', 'EnergyRemaining','Startbit', [ 0;],'SignalSize', [ 16;],'ByteOrder', 'LittleEndian','ValueType', 'UNSIGNED','Class', 'uint16','Signed', [ 0;],'Factor', [ 0.005;],'Offset', [ 0;],'Min', [ 0;],'Max', [ 0;],'Units', 'kWh','Comment', 'Energy remaining until the battery pack reaches 0% state of charge.','StartBit', [ 0;])}}
      settings: SourceProductName=Raptor
  Data : Outport  VectorParamsAs1DForOutWhenUnconnected=off
  wires:
  Bus Creator/1 -> Data/1  "BMS6_Energy"
  raptor_can_rxmsg/2 -> CANRxField1/1  "Batt_EnergyRemaining"
  CANRxField1/1 -> Bus Creator/2
  CANRxMsgStatus/1 -> Bus Creator/1
  DiagEnbl/1 -> CANRxMsgStatus/1
  raptor_can_rxmsg/1 -> CANRxMsgStatus/2  "Age"

== system VCMGCM1962020b_v2/Fgnd/Sensors/CAN/Battery/BMS7_Diagnostics ==
  DiagEnbl : Inport
  Bus Creator : BusCreator  Inputs=2
  CANRxField1 : Blocks_lib/CANRxField  typ='double'  custom=off  custom_nam='---'  custom_units='---'
  CANRxMsgStatus : Blocks_lib/CANRxMsgStatus  samptime=samptime  custom=off  custom_nam='---'  msgnam=BMS7_Diagnostics
      link override CntrSat/Constant: OutDataTypeStr=uint32
      link override CntrSat/Constant1: OutDataTypeStr=uint32
      link override CntrSat/Relational Operator: Operator=>
      link override CntrSat/raptor_adjustment: dataType=uint32
  Header : Blocks_lib/Header  width=Landscape  addtext=''
  raptor_can_rxmsg : Raptor_lib/CAN/raptor_can_rxmsg  canDefinition=struct('dbcFile', 'eMatrix_Battery.dbc','message', 'BMS7_Diagnostics','comment', '','signals', {{'V_BAT','T_Cell_Min','T_Cell_Max','V_Cell_Min','V_Cell_Max'}},'enabled', [ 1 1 1 1 1;],'scaled', [ 1 1 1 1 1;],'canBus', '''CAN1''','messageID', [ 1808;],'idMask', [ 536870911;],'payloadMask', [],'payloadValue', [],'period', [ 0;],'mailbox', '''''','queueSize', [ 1;],'label', [ 0;],'ver', [ 2;],'showID', [ 0;],'showRaw', [ 0;],'fill', [ 0;],'editID', [ 0;],'signalOrder', [ 3;],'signalAscDes', [ 1;])  canBus='CAN1'  mailbox=''  payloadMask=[]  payloadValue=[]  idMask=hex2dec('1FFFFFFF')  queueSize=1  showID=0  label=0  fill=0  id=1808  showRaw=0  showAge=1  signalOrder=3  signalInfo={{struct('Name', 'V_BAT','Startbit', [ 0;],'SignalSize', [ 16;],'ByteOrder', 'LittleEndian','ValueType', 'UNSIGNED','Class', 'uint16','Signed', [ 0;],'Factor', [ 0.1;],'Offset', [ 0;],'Min', [ 0;],'Max', [ 450;],'Units', 'V','Comment', 'Total Battery Voltage','StartBit', [ 48;]),struct('Name', 'T_Cell_Min','Startbit', [ 0;],'SignalSize', [ 8;],'ByteOrder', 'LittleEndian','ValueType', 'UNSIGNED','Class', 'uint8','Signed', [ 0;],'Factor', [ 0.5;],'Offset', [ -40;],'Min', [ -40;],'Max', [ 87.5;],'Units', 'C','Comment', 'Minimum Cell Temperature','StartBit', [ 40;]),struct('Name', 'T_Cell_Max','Startbit', [ 0;],'SignalSize', [ 8;],'ByteOrder', 'LittleEndian','ValueType', 'UNSIGNED','Class', 'uint8','Signed', [ 0;],'Factor', [ 0.5;],'Offset', [ -40;],'Min', [ -40;],'Max', [ 87.5;],'Units', 'C','Comment', 'Maximum cell Temperature','StartBit', [ 32;]),struct('Name', 'V_Cell_Min','Startbit', [ 0;],'SignalSize', [ 16;],'ByteOrder', 'LittleEndian','ValueType', 'UNSIGNED','Class', 'uint16','Signed', [ 0;],'Factor', [ 0.001;],'Offset', [ 0;],'Min', [ 0;],'Max', [ 10;],'Units', 'V','Comment', 'Instantaneous minimum cell voltage.','StartBit', [ 16;]),struct('Name', 'V_Cell_Max','Startbit', [ 0;],'SignalSize', [ 16;],'ByteOrder', 'LittleEndian','ValueType', 'UNSIGNED','Class', 'uint16','Signed', [ 0;],'Factor', [ 0.001;],'Offset', [ 0;],'Min', [ 0;],'Max', [ 10;],'Units', 'V','Comment', 'Instantaneous maximum Cell voltage.','StartBit', [ 0;])}}
      settings: SourceProductName=Raptor
  Data : Outport  VectorParamsAs1DForOutWhenUnconnected=off
  wires:
  Bus Creator/1 -> Data/1  "MsgName"
  CANRxField1/1 -> Bus Creator/2
  CANRxMsgStatus/1 -> Bus Creator/1
  DiagEnbl/1 -> CANRxMsgStatus/1
  raptor_can_rxmsg/1 -> CANRxMsgStatus/2  "Age"

== system VCMGCM1962020b_v2/Fgnd/Sensors/CAN/Battery/Batt_Pack_Cell_Voltage_Stats ==
  DiagEnbl : Inport
  Bus Creator : BusCreator  Inputs=5
  CANRxField{,1..3} (4 alike) : Blocks_lib/CANRxField  typ='double'  custom=off  custom_nam='---'  custom_units='---'
  CANRxMsgStatus : Blocks_lib/CANRxMsgStatus  samptime=samptime  custom=off  custom_nam='Name'  msgnam=Batt_Pack_Cell_Voltage_Stats
  Header : Blocks_lib/Header  width=Landscape  addtext=''
  raptor_can_rxmsg : Raptor_lib/CAN/raptor_can_rxmsg  canDefinition=struct('dbcFile', 'BMS dbc file_rev6.0.dbc','message', 'Batt_Pack_Cell_Voltage_Stats','comment', '','signals', {{'Batt_Pack0_Min_Volt','Batt_Pack0_Max_Volt','Batt_Pack1_Min_Volt','Batt_Pack1_Max_Volt'}},'enabled', [ 1 1 1 1;],'scaled', [ 1 1 1 1;],'canBus', 'bus','messageID', [ 218040307;],'idMask', [ 536870911;],'payloadMask', [],'payloadValue', [],'period', [ 0;],'mailbox', '''''','queueSize', [ 1;],'label', [ 1;],'ver', [ 2;],'showID', [ 0;],'showRaw', [ 0;],'fill', [ 0;],'editID', [ 0;],'signalOrder', [ 3;],'signalAscDes', [ 1;])  canBus=bus  mailbox=''  payloadMask=[]  payloadValue=[]  idMask=hex2dec('1FFFFFFF')  queueSize=1  showID=0  label=1  fill=0  id=218040307  showRaw=0  showAge=1  signalOrder=3  signalInfo={{struct('Name', 'Batt_Pack0_Min_Volt','Startbit', [ 0;],'SignalSize', [ 16;],'ByteOrder', 'LittleEndian','ValueType', 'UNSIGNED','Class', 'uint16','Signed', [ 0;],'Factor', [ 0.1;],'Offset', [ 0;],'Min', [ 0;],'Max', [ 0;],'Units', 'V','Comment', '','StartBit', [ 0;]),struct('Name', 'Batt_Pack0_Max_Volt','Startbit', [ 0;],'SignalSize', [ 16;],'ByteOrder', 'LittleEndian','ValueType', 'UNSIGNED','Class', 'uint16','Signed', [ 0;],'Factor', [ 0.1;],'Offset', [ 0;],'Min', [ 0;],'Max', [ 0;],'Units', 'V','Comment', '','StartBit', [ 16;]),struct('Name', 'Batt_Pack1_Min_Volt','Startbit', [ 0;],'SignalSize', [ 16;],'ByteOrder', 'LittleEndian','ValueType', 'UNSIGNED','Class', 'uint16','Signed', [ 0;],'Factor', [ 0.1;],'Offset', [ 0;],'Min', [ 0;],'Max', [ 0;],'Units', 'V','Comment', '','StartBit', [ 32;]),struct('Name', 'Batt_Pack1_Max_Volt','Startbit', [ 0;],'SignalSize', [ 16;],'ByteOrder', 'LittleEndian','ValueType', 'UNSIGNED','Class', 'uint16','Signed', [ 0;],'Factor', [ 0.1;],'Offset', [ 0;],'Min', [ 0;],'Max', [ 0;],'Units', 'V','Comment', '','StartBit', [ 48;])}}
      settings: SourceProductName=Raptor
  Data : Outport  VectorParamsAs1DForOutWhenUnconnected=off
  wires:
  Bus Creator/1 -> Data/1  "MsgName"
  raptor_can_rxmsg/2 -> CANRxField/1  "Batt_Pack0_Min_Volt"
  CANRxMsgStatus/1 -> Bus Creator/1
  CANRxField/1 -> Bus Creator/2
  DiagEnbl/1 -> CANRxMsgStatus/1
  raptor_can_rxmsg/1 -> CANRxMsgStatus/2  "Age"
  raptor_can_rxmsg/5 -> CANRxField3/1  "Batt_Pack1_Max_Volt"
  raptor_can_rxmsg/3 -> CANRxField1/1  "Batt_Pack0_Max_Volt"
  raptor_can_rxmsg/4 -> CANRxField2/1  "Batt_Pack1_Min_Volt"
  CANRxField1/1 -> Bus Creator/3
  CANRxField2/1 -> Bus Creator/4
  CANRxField3/1 -> Bus Creator/5

== system VCMGCM1962020b_v2/Fgnd/Sensors/CAN/Battery/Command ==
  DiagEnbl : Inport
  Bus Creator : BusCreator  Inputs=5
  CANRxField1 : Blocks_lib/CANRxField  typ='double'  custom=off  custom_nam='---'  custom_units='---'
  CANRxField2 : Blocks_lib/CANRxField  typ='uint8'  custom=off  custom_nam='---'  custom_units='---'
  CANRxField3 : Blocks_lib/CANRxField  typ='boolean'  custom=off  custom_nam='---'  custom_units='---'
  CANRxField4 : Blocks_lib/CANRxField  typ='boolean'  custom=off  custom_nam='---'  custom_units='---'
  CANRxMsgStatus : Blocks_lib/CANRxMsgStatus  samptime=samptime  custom=off  custom_nam='---'  msgnam=Command
      link override CntrSat/Constant: OutDataTypeStr=uint32
      link override CntrSat/Constant1: OutDataTypeStr=uint32
      link override CntrSat/Relational Operator: Operator=>
      link override CntrSat/raptor_adjustment: dataType=uint32
  Header : Blocks_lib/Header  width=Landscape  addtext=''
  raptor_can_rxmsg : Raptor_lib/CAN/raptor_can_rxmsg  canDefinition=struct('dbcFile', 'eMatrix_Battery.dbc','message', 'Command','comment', '','signals', {{'TestMode','ChargeMode','DisableGFD','MainContactorRequest'}},'enabled', [ 1 1 1 1;],'scaled', [ 1 1 1 1;],'canBus', '''CAN1''','messageID', [ 272;],'idMask', [ 536870911;],'payloadMask', [],'payloadValue', [],'period', [ 0;],'mailbox', '''''','queueSize', [ 1;],'label', [ 0;],'ver', [ 2;],'showID', [ 0;],'showRaw', [ 0;],'fill', [ 0;],'editID', [ 0;],'signalOrder', [ 3;],'signalAscDes', [ 1;])  canBus='CAN1'  mailbox=''  payloadMask=[]  payloadValue=[]  idMask=hex2dec('1FFFFFFF')  queueSize=1  showID=0  label=0  fill=0  id=272  showRaw=0  showAge=1  signalOrder=3  signalInfo={{struct('Name', 'TestMode','Startbit', [ 0;],'SignalSize', [ 1;],'ByteOrder', 'LittleEndian','ValueType', 'UNSIGNED','Class', 'uint8','Signed', [ 0;],'Factor', [ 1;],'Offset', [ 0;],'Min', [ 0;],'Max', [ 0;],'Units', '','Comment', '0 = False','StartBit', [ 16;]),struct('Name', 'ChargeMode','Startbit', [ 0;],'SignalSize', [ 1;],'ByteOrder', 'LittleEndian','ValueType', 'UNSIGNED','Class', 'uint8','Signed', [ 0;],'Factor', [ 1;],'Offset', [ 0;],'Min', [ 0;],'Max', [ 0;],'Units', '','Comment', '0 = Drive Mode','StartBit', [ 1;]),struct('Name', 'DisableGFD','Startbit', [ 0;],'SignalSize', [ 8;],'ByteOrder', 'LittleEndian','ValueType', 'UNSIGNED','Class', 'uint8','Signed', [ 0;],'Factor', [ 1;],'Offset', [ 0;],'Min', [ 0;],'Max', [ 0;],'Units', '','Comment', '1 = Disable Ground Fault Detection','StartBit', [ 8;]),struct('Name', 'MainContactorRequest','Startbit', [ 0;],'SignalSize', [ 1;],'ByteOrder', 'LittleEndian','ValueType', 'UNSIGNED','Class', 'uint8','Signed', [ 0;],'Factor', [ 1;],'Offset', [ 0;],'Min', [ 0;],'Max', [ 0;],'Units', '','Comment', '0 = Open','StartBit', [ 0;])}}
      settings: SourceProductName=Raptor
  Data : Outport  VectorParamsAs1DForOutWhenUnconnected=off
  wires:
  Bus Creator/1 -> Data/1  "Command"
  CANRxField2/1 -> Bus Creator/3
  CANRxField3/1 -> Bus Creator/4
  CANRxField4/1 -> Bus Creator/5
  raptor_can_rxmsg/2 -> CANRxField1/1  "Var51"
  raptor_can_rxmsg/3 -> CANRxField2/1  "Var52"
  raptor_can_rxmsg/4 -> CANRxField3/1  "Var53"
  raptor_can_rxmsg/5 -> CANRxField4/1  "Var54"
  CANRxField1/1 -> Bus Creator/2
  CANRxMsgStatus/1 -> Bus Creator/1
  DiagEnbl/1 -> CANRxMsgStatus/1
  raptor_can_rxmsg/1 -> CANRxMsgStatus/2  "Age"
